simulink model "Lasermeltpool_controller_simulink_design_1"  (R2019a)
settings: Solver=VariableStepAuto  StartTime=0.0  StopTime=10  RelTol=1e-3
libraries: simulink x6, slident x2, cstblocks x1, robotcorelib x1
settings Model: Creator=MI  LastModifiedBy=MI

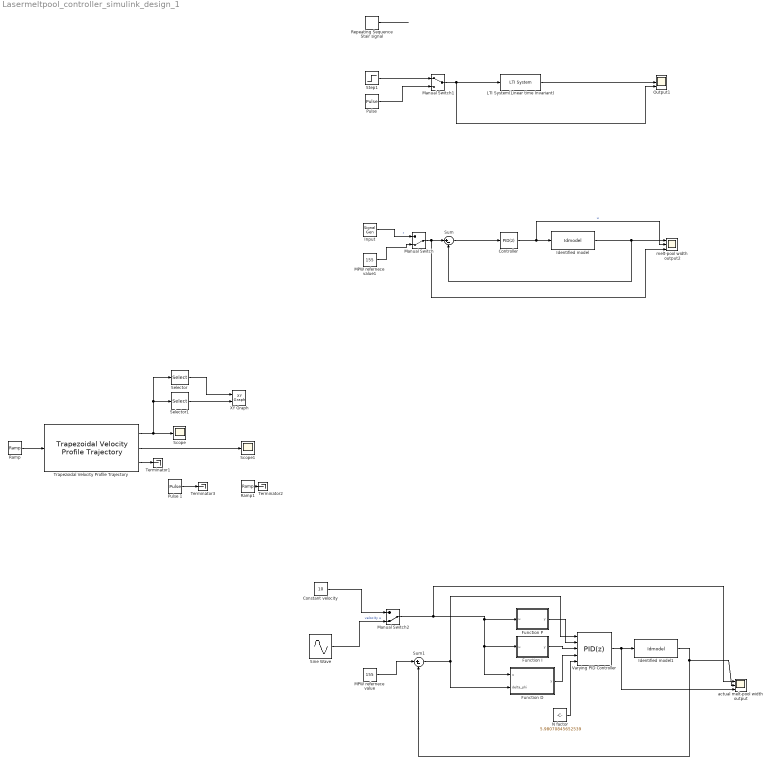
== system Lasermeltpool_controller_simulink_design_1 ==
  Constant velocity : Constant  Value=10
  Controller : simulink/Continuous/PID Controller  Controller=PID  Form=Parallel  TimeDomain=Discrete-time  SampleTime=-1  IntegratorMethod=Forward Euler  FilterMethod=Forward Euler  ControllerParametersSource=internal  P=0.000563720445923274  I=0.0341648755105015  D=0  UseFilter=on  N=100  TunerSelectOption=Transfer Function Based (PID Tuner App)  InitialConditionSource=internal  InitialConditionForIntegrator=0  InitialConditionForFilter=0  DifferentiatorICPrevScaledInput=0  ExternalReset=none  TrackingMode=off  Kt=1  LimitOutput=off  UpperSaturationLimit=inf  LowerSaturationLimit=-inf  LinearizeAsGain=on  AntiWindupMode=none  Kb=1  POutMin=[]  POutMax=[]  IOutMin=[]  IOutMax=[]  DOutMin=[]  DOutMax=[]  NOutMin=[]  NOutMax=[]  SumOutMin=[]  SumOutMax=[]  SaturationOutMin=[]  SaturationOutMax=[]  PParamMin=[]  PParamMax=[]  IParamMin=[]  IParamMax=[]  DParamMin=[]  DParamMax=[]  NParamMin=[]  NParamMax=[]  KbParamMin=[]  KbParamMax=[]  KtParamMin=[]  KtParamMax=[]  KbOutMin=[]  KbOutMax=[]  KtOutMin=[]  KtOutMax=[]  IntegratorOutMin=[]  IntegratorOutMax=[]  FilterOutMin=[]  FilterOutMax=[]  SumI1OutMin=[]  SumI1OutMax=[]  SumI2OutMin=[]  SumI2OutMax=[]  SumI3OutMin=[]  SumI3OutMax=[]  SumI4OutMin=[]  SumI4OutMax=[]  SumDOutMin=[]  SumDOutMax=[]  DifferentiatorOutMin=[]  DifferentiatorOutMax=[]  FilterDiffOutCoefMin=[]  FilterDiffOutCoefMax=[]  ReciprocalOutMin=[]  ReciprocalOutMax=[]  SumDenOutMin=[]  SumDenOutMax=[]  SumNumOutMin=[]  SumNumOutMax=[]  DivideOutMin=[]  DivideOutMax=[]  IntegratorContinuousStateAttributes=''  IntegratorStateMustResolveToSignalObject=off  IntegratorRTWStateStorageClass=Auto  FilterContinuousStateAttributes=''  FilterStateMustResolveToSignalObject=off  FilterRTWStateStorageClass=Auto  ParallelPVariant=InternalParameters  IdealPVariant=Disabled  IVariant=InternalParameters  DVariant=InternalParameters  IntegratorVariant=Discrete  SatVariant=Disabled  AWVariant=Passthrough  PCopyVariant=Disabled  TRVariant=Disabled  FdbkBlocksVariant=Forward  IdealPFdbkVariant=Disabled  SatFdbkVariant=Disabled  DerivativeFilterVariant=ForwardEulerFilter  NVariant=InternalParameters  NCopyVariant=Disabled  FilterICVariant=InternalICsFilter  IntegratorICVariant=InternalICs  ExternalResetVariant=Disabled  TRSumVariant=Passthrough  SumFdbkVariant=Disabled  SumVariant=Sum_PID
  Function D : MATLAB Function  TreatAsAtomicUnit=on
  Function I : MATLAB Function  TreatAsAtomicUnit=on
  Function P : MATLAB Function  TreatAsAtomicUnit=on
  Identified model : slident/Models/Idmodel  sys=Plant1  IC=0  noi=off  seed=[]
      settings: SourceProductBaseCode=ID
  Identified model1 : slident/Models/Idmodel  sys=Plant1  IC=0  noi=off  seed=[]
      settings: SourceProductBaseCode=ID
  Input : SignalGenerator
  LTI System(Linear time Invariant) : cstblocks/LTI System  sys=Plant1  IC=[]
  MPW refernece value : Constant  Value=155
  MPW refernece value1 : Constant  Value=155
  Manual Switch : ManualSwitch  CurrentSetting=0
  Manual Switch1 : ManualSwitch
  Manual Switch2 : ManualSwitch  CurrentSetting=0
  N factor : Constant  Value=5.98070845652539
  Output1 : Scope  NumInputPorts=3
  "Pulse " : DiscretePulseGenerator  PulseType=Time based  Amplitude=3.8  Period=10  PulseWidth=5
  Pulse 1 : DiscretePulseGenerator  PulseType=Time based  Amplitude=10  Period=10  PulseWidth=95
  Ramp : simulink/Sources/Ramp  slope=1  start=0  InitialOutput=0
  Ramp1 : simulink/Sources/Ramp  slope=10  start=0  InitialOutput=0
  Repeating Sequence Stair signal : simulink/Sources/Repeating Sequence Stair  OutValues=[3 1 4 2 1].'  tsamp=-1  OutMin=[]  OutMax=[]  OutDataTypeStr=double  OutputDataTypeScalingMode=double  OutDataType=fixdt(0,8)  ConRadixGroup=Best Precision: Vector-wise  OutScaling=2^-12
  Scope : Scope
  Scope1 : Scope
  Selector : Selector  InputPortWidth=2  IndexOptions=Index vector (dialog)  Indices=1  OutputSizes=1
  Selector1 : Selector  InputPortWidth=2  IndexOptions=Index vector (dialog)  Indices=2  OutputSizes=1
  Sine Wave : Sin  Amplitude=0.1  Bias=10  Frequency=20  SampleTime=0.033
  Step1 : Step  After=3.8  SampleTime=0
  Sum : Sum  Inputs=|+-
  Sum1 : Sum  Inputs=|+-
  Terminator1 : Terminator
  Terminator2 : Terminator
  Terminator3 : Terminator
  Trapezoidal Velocity Profile Trajectory : robotcorelib/Trapezoidal Velocity Profile Trajectory  WaypointSource=Internal  Waypoints=[ 0, -0.5, -1, 1; 0, 0.5, 1, 1]  NumParams=0  Parameter1=Peak Velocity  Parameter2=End Time  ParameterSource=Internal  PeakVelocity=[ 2; 2 ]  Acceleration=[ 1; 2 ]  EndTime=[ 1; 1 ]  AccelTime=[ 1; 2 ]  SimulateUsing=Interpreted execution
      settings: SourceProductName=Robotics System Toolbox  SourceProductBaseCode=RO
  Varying PID Controller : simulink/Continuous/PID Controller  Controller=PID  Form=Parallel  TimeDomain=Discrete-time  SampleTime=-1  IntegratorMethod=Forward Euler  FilterMethod=Forward Euler  ControllerParametersSource=external  P=1  I=1  D=0  UseFilter=on  N=100  TunerSelectOption=Transfer Function Based (PID Tuner App)  InitialConditionSource=internal  InitialConditionForIntegrator=0  InitialConditionForFilter=0  DifferentiatorICPrevScaledInput=0  ExternalReset=none  TrackingMode=off  Kt=1  LimitOutput=off  UpperSaturationLimit=inf  LowerSaturationLimit=-inf  LinearizeAsGain=on  AntiWindupMode=none  Kb=1  POutMin=[]  POutMax=[]  IOutMin=[]  IOutMax=[]  DOutMin=[]  DOutMax=[]  NOutMin=[]  NOutMax=[]  SumOutMin=[]  SumOutMax=[]  SaturationOutMin=[]  SaturationOutMax=[]  PParamMin=[]  PParamMax=[]  IParamMin=[]  IParamMax=[]  DParamMin=[]  DParamMax=[]  NParamMin=[]  NParamMax=[]  KbParamMin=[]  KbParamMax=[]  KtParamMin=[]  KtParamMax=[]  KbOutMin=[]  KbOutMax=[]  KtOutMin=[]  KtOutMax=[]  IntegratorOutMin=[]  IntegratorOutMax=[]  FilterOutMin=[]  FilterOutMax=[]  SumI1OutMin=[]  SumI1OutMax=[]  SumI2OutMin=[]  SumI2OutMax=[]  SumI3OutMin=[]  SumI3OutMax=[]  SumI4OutMin=[]  SumI4OutMax=[]  SumDOutMin=[]  SumDOutMax=[]  DifferentiatorOutMin=[]  DifferentiatorOutMax=[]  FilterDiffOutCoefMin=[]  FilterDiffOutCoefMax=[]  ReciprocalOutMin=[]  ReciprocalOutMax=[]  SumDenOutMin=[]  SumDenOutMax=[]  SumNumOutMin=[]  SumNumOutMax=[]  DivideOutMin=[]  DivideOutMax=[]  IntegratorContinuousStateAttributes=''  IntegratorStateMustResolveToSignalObject=off  IntegratorRTWStateStorageClass=Auto  FilterContinuousStateAttributes=''  FilterStateMustResolveToSignalObject=off  FilterRTWStateStorageClass=Auto  ParallelPVariant=ExternalParameters  IdealPVariant=Disabled  IVariant=ExternalParameters  DVariant=ExternalParameters  IntegratorVariant=Discrete  SatVariant=Disabled  AWVariant=Passthrough  PCopyVariant=Disabled  TRVariant=Disabled  FdbkBlocksVariant=Forward  IdealPFdbkVariant=Disabled  SatFdbkVariant=Disabled  DerivativeFilterVariant=ForwardEulerFilter  NVariant=ExternalParameters  NCopyVariant=Disabled  FilterICVariant=InternalICsFilter  IntegratorICVariant=InternalICs  ExternalResetVariant=Disabled  TRSumVariant=Passthrough  SumFdbkVariant=Disabled  SumVariant=Sum_PID
  XY Graph : simulink/Sinks/XY Graph  xmin=-3  xmax=5  ymin=-1  ymax=5  st=-1
  actual melt-pool width output : Scope  NumInputPorts=3
  melt-pool width output2 : Scope  NumInputPorts=3
  wires:
  Manual Switch/1 -> melt-pool width output2/3, Sum/1
  Sum/1 -> Controller/1
  Controller/1 -> melt-pool width output2/2, Identified model/1  "u"
  MPW refernece value1/1 -> Manual Switch/2
  "Pulse "/1 -> Manual Switch1/2
  Identified model/1 -> Sum/2, melt-pool width output2/1
  LTI System(Linear time Invariant)/1 -> Output1/2
  Step1/1 -> Manual Switch1/1
  Manual Switch1/1 -> Output1/3, LTI System(Linear time Invariant)/1
  Identified model1/1 -> Sum1/2, actual melt-pool width output/2
  Varying PID Controller/1 -> Identified model1/1, actual melt-pool width output/3
  Function P/1(y) -> Varying PID Controller/2
  Function I/1(y) -> Varying PID Controller/3
  Function D/1(y) -> Varying PID Controller/4
  Sum1/1 -> Varying PID Controller/1, Function D/2(delta_phi)
  MPW refernece value/1 -> Sum1/1
  Manual Switch2/1 -> actual melt-pool width output/1, Function D/1(u), Function I/1(u), Function P/1(u)
  N factor/1 -> Varying PID Controller/5
  Sine Wave/1 -> Manual Switch2/2  "velocity u"
  Input/1 -> Manual Switch/1  "r"
  Repeating Sequence Stair signal/1 -> ?
  Selector/1 -> XY Graph/1
  Trapezoidal Velocity Profile Trajectory/2 -> Scope1/1
  Ramp/1 -> Trapezoidal Velocity Profile Trajectory/1
  Trapezoidal Velocity Profile Trajectory/1 -> Selector1/1, Selector/1, Scope/1
  Trapezoidal Velocity Profile Trajectory/3 -> Terminator1/1
  Selector1/1 -> XY Graph/2
  Constant velocity/1 -> Manual Switch2/1
  Pulse 1/1 -> Terminator3/1
  Ramp1/1 -> Terminator2/1

== matlab function Lasermeltpool_controller_simulink_design_1/Function I ==
  data: u input; y output
function y = fcn(u)

% I control action: eliminates steady states error, but will result
% oscillarity 

Ki0 = 0.0341648755105015; % nominal value of Ki

y = Ki0;


end

== matlab function Lasermeltpool_controller_simulink_design_1/Function P ==
  data: u input; y output
function y = fcn(u)

%This function calculates the required P parameters
% according to the speed, u is speed here y is the output of calculation

Kp0 = 0.000563720445923274; % this is the nominal value of Kp gain， 
                          % which is get from pid tuning process
u0 = 10; % nominal value of the speed 
y = Kp0; % assign output to the Kp0 as defult

alpha = 0.00033; % coefficient of P parameter change 
if(u > u0) % if speed is faster than nominal, brings more uncertainty to meltpool dynamics.
    % P control action will increase response speed but higher noise
    % sensitivity and instability, therefore, reduce p parameter here
    y = Kp0 - alpha * (u-u0);
end 

if(u < u0)
    y = Kp0 + alpha * (u0-u);
end

end

== matlab function Lasermeltpool_controller_simulink_design_1/Function D ==
  data: u input; y output; delta_phi input
function y = fcn(u, delta_phi)
% D control action: improve stability, increase damping(decrease
% oscillation), sensitive to noise. imporve transient response. 

Kd0 = -0.000108487487850706; % norminal Kd gain
u0 = 10;
alpha = 0.0003; % coefficient of Kd changing

Kd = Kd0;

if (u > u0) 
    if (delta_phi > 0)
        % decrease power, with Kd gain inversly propotional to speed change
        Kd = Kd0 + alpha / (u-u0); 
    end
    if (delta_phi < 0)
        % increase power, with Kd gain propotional to speed change
        Kd = Kd0 + alpha * (u-u0); 
    end
end

if (u < u0) 
    if (delta_phi > 0)
        % decrease power, with Kd gain inversly propotional to speed change
        Kd = Kd0 + alpha * (u0-u); 
    end
    if (delta_phi < 0)
        % decrease power, with Kd gain inversly propotional to speed change
        Kd = Kd0 + alpha / (u0-u); 
    end
end


y = Kd


end
